simulink model "chris_4R_all_primitives"  (R2024b)
settings: Solver=FixedStepDiscrete  StartTime=0.0  StopTime=60  FixedStep=0.1  MaxStep=0.1  RelTol=1e-3
libraries: neural x220, simulink x1, realtime_pacer_lib x1
(part 1 of 9)
settings Model: Creator=RSL  LastModifiedBy=cwaight
settings SolverCC: AlgebraicLoopSolver=TrustRegion
settings DataIOCC: ReturnWorkspaceOutputs=off
settings DebuggingCC: UnconnectedInputMsg=warning  UnconnectedOutputMsg=warning  UnconnectedLineMsg=warning  ArithmeticOperatorsInVariantConditions=warning
settings ModelReferenceCC: EnableRefExpFcnMdlSchedulingChecks=on
settings SFSimCC: SimUseLocalCustomCode=off  CustomCodeUndefinedFunction=UseInterfaceOnly
settings RTWCC: RTWUseLocalCustomCode=off  GPUComputeCapability=3.5
settings CodeAppCC: StateflowObjectComments=on

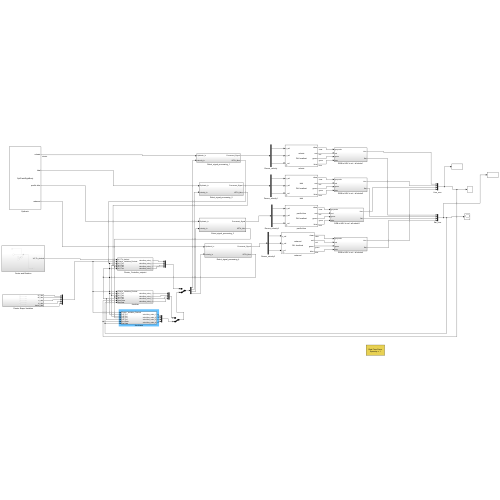
[thumbnail: Simulink's stored preview of the top-level diagram]
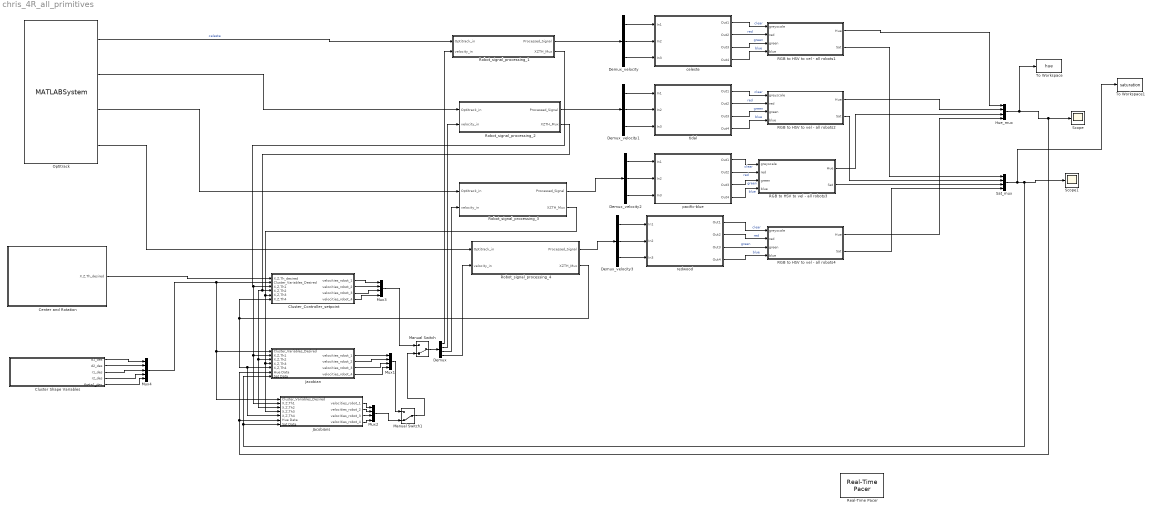
== system chris_4R_all_primitives ==
  Center and Rotation : Subsystem
  Cluster Shape Variables : Subsystem
  Cluster_Controller_setpoint : Subsystem
  Demux : Demux
  Demux_velocity{,1..3} (4 alike) : Demux  Outputs=3
  Hue_mux : Mux
  Jacobian : Subsystem
  Jacobians : Subsystem
  Manual Switch : ManualSwitch  CurrentSetting=0
  Manual Switch1 : ManualSwitch  CurrentSetting=0
  Mux1 : Mux
  Mux2 : Mux
  Mux3 : Mux
  Mux4 : Mux  Inputs=5
  Optitrack : MATLABSystem  System=OptiTrackRigidBody  coordinateTransformationMatrix=[ 1, 0, 0; 0, 0, 1; 0, -1, 0 ]  rigidBodyNames={ 'celeste','tidal','pacific-blue','redwood'}  orientationFormat=Euler angles  debug=on  natNetHostAddress=127.0.0.1  natNetClientAddress=127.0.0.1  dllPath=C:\DecaMATLAB\NatNetSDK\lib\x64\NatNetML.dll  unicast=off
      mask Type: OptiTrackRigidBody
      mask Display:
      | disp('OptiTrackRigidBody');
      | port_label('output',1,'celeste');
      | port_label('output',2,'tidal');
      | port_label('output',3,'pacific-blue');
      | port_label('output',4,'redwood');
  RGB to HSV to vel - all robots1 : Subsystem
  RGB to HSV to vel - all robots2 : Subsystem
  RGB to HSV to vel - all robots3 : Subsystem
  RGB to HSV to vel - all robots4 : Subsystem
  Real-Time Pacer : realtime_pacer_lib/Real-Time Pacer  simTimePerRealTime=1
  Robot_signal_processing_1 : Subsystem
  Robot_signal_processing_2 : Subsystem
  Robot_signal_processing_3 : Subsystem
  Robot_signal_processing_4 : Subsystem
  Sat_mux : Mux
  Scope : Scope
  Scope1 : Scope
  To Workspace : ToWorkspace  VariableName=hue  SaveFormat=Timeseries  SampleTime=-1
  To Workspace1 : ToWorkspace  VariableName=saturation  SaveFormat=Timeseries  SampleTime=-1
  celeste : Subsystem  mask(DecabotMask){robotName=celeste, decabotHelper=localhost, robotAddress=, useDataTurbine=off, useDirectSocket=on, debug=off}
      mask prompts: robotName "Robot name:"; decabotHelper "DecabotHelper/DataTurbine server:"; robotAddress "Robot network address (optional):"; useDataTurbine "Use DataTurbine"; useDirectSocket "Use direct robot TCP connection"; debug "Log debug messages"
      mask help: This is a masked subsystem that contains a Decabot block for bidirectional communication with a decabot over a direct TCP socket connection.
      mask init:
      | robotName = 'Nobody';
      | decabotHelper = 'localhost';
      | robotAddress = '';
      | useDataTurbine = true;
      | debug = true;
      mask TypeOptions robotName: decabot/robotName
      mask Callback robotName:
      | try
      |     set_param( gcb( ), 'Name', get_param( gcb( ), 'robotName' ) );
      | end
      mask TypeOptions decabotHelper: decabot/decabotHelper
      mask TypeOptions robotAddress: decabot/robotAddress
      mask TypeOptions useDataTurbine: decabot/useDataTurbine
      mask TypeOptions useDirectSocket: decabot/useDirectSocket
      mask TypeOptions debug: decabot/debug
      mask Display:
      | disp( [get_param( gcb( ), 'robotName' ) '\n\nDH: ' get_param( gcb( ), 'decabotHelper' ) ] );
      | 
      | port_label('input',1,'x_vel');
      | port_label('input',2,'y_vel');
      | port_label('input',3,'t_vel');
      | 
      | port_label('output',1,'clear');
      | port_label('output',2,'red');
      | port_label('output',3,'green');
      | port_label('output',4,'blue');
  pacific-blue : Subsystem  mask(DecabotMask){robotName=pacific-blue, decabotHelper=localhost, robotAddress=, useDataTurbine=off, useDirectSocket=on, debug=off}
      mask prompts: robotName "Robot name:"; decabotHelper "DecabotHelper/DataTurbine server:"; robotAddress "Robot network address (optional):"; useDataTurbine "Use DataTurbine"; useDirectSocket "Use direct robot TCP connection"; debug "Log debug messages"
      mask help: This is a masked subsystem that contains a Decabot block for bidirectional communication with a decabot over a direct TCP socket connection.
      mask init:
      | robotName = 'Nobody';
      | decabotHelper = 'localhost';
      | robotAddress = '';
      | useDataTurbine = true;
      | debug = true;
      mask TypeOptions robotName: decabot/robotName
      mask Callback robotName:
      | try
      |     set_param( gcb( ), 'Name', get_param( gcb( ), 'robotName' ) );
      | end
      mask TypeOptions decabotHelper: decabot/decabotHelper
      mask TypeOptions robotAddress: decabot/robotAddress
      mask TypeOptions useDataTurbine: decabot/useDataTurbine
      mask TypeOptions useDirectSocket: decabot/useDirectSocket
      mask TypeOptions debug: decabot/debug
      mask Display:
      | disp( [get_param( gcb( ), 'robotName' ) '\n\nDH: ' get_param( gcb( ), 'decabotHelper' ) ] );
      | 
      | port_label('input',1,'x_vel');
      | port_label('input',2,'y_vel');
      | port_label('input',3,'t_vel');
      | 
      | port_label('output',1,'clear');
      | port_label('output',2,'red');
      | port_label('output',3,'green');
      | port_label('output',4,'blue');
  redwood : Subsystem  mask(DecabotMask){robotName=redwood, decabotHelper=localhost, robotAddress=, useDataTurbine=off, useDirectSocket=on, debug=off}
      mask prompts: robotName "Robot name:"; decabotHelper "DecabotHelper/DataTurbine server:"; robotAddress "Robot network address (optional):"; useDataTurbine "Use DataTurbine"; useDirectSocket "Use direct robot TCP connection"; debug "Log debug messages"
      mask help: This is a masked subsystem that contains a Decabot block for bidirectional communication with a decabot over a direct TCP socket connection.
      mask init:
      | robotName = 'Nobody';
      | decabotHelper = 'localhost';
      | robotAddress = '';
      | useDataTurbine = true;
      | debug = true;
      mask TypeOptions robotName: decabot/robotName
      mask Callback robotName:
      | try
      |     set_param( gcb( ), 'Name', get_param( gcb( ), 'robotName' ) );
      | end
      mask TypeOptions decabotHelper: decabot/decabotHelper
      mask TypeOptions robotAddress: decabot/robotAddress
      mask TypeOptions useDataTurbine: decabot/useDataTurbine
      mask TypeOptions useDirectSocket: decabot/useDirectSocket
      mask TypeOptions debug: decabot/debug
      mask Display:
      | disp( [get_param( gcb( ), 'robotName' ) '\n\nDH: ' get_param( gcb( ), 'decabotHelper' ) ] );
      | 
      | port_label('input',1,'x_vel');
      | port_label('input',2,'y_vel');
      | port_label('input',3,'t_vel');
      | 
      | port_label('output',1,'clear');
      | port_label('output',2,'red');
      | port_label('output',3,'green');
      | port_label('output',4,'blue');
  tidal : Subsystem  mask(DecabotMask){robotName=tidal, decabotHelper=localhost, robotAddress=, useDataTurbine=off, useDirectSocket=on, debug=off}
      mask prompts: robotName "Robot name:"; decabotHelper "DecabotHelper/DataTurbine server:"; robotAddress "Robot network address (optional):"; useDataTurbine "Use DataTurbine"; useDirectSocket "Use direct robot TCP connection"; debug "Log debug messages"
      mask help: This is a masked subsystem that contains a Decabot block for bidirectional communication with a decabot over a direct TCP socket connection.
      mask init:
      | robotName = 'Nobody';
      | decabotHelper = 'localhost';
      | robotAddress = '';
      | useDataTurbine = true;
      | debug = true;
      mask TypeOptions robotName: decabot/robotName
      mask Callback robotName:
      | try
      |     set_param( gcb( ), 'Name', get_param( gcb( ), 'robotName' ) );
      | end
      mask TypeOptions decabotHelper: decabot/decabotHelper
      mask TypeOptions robotAddress: decabot/robotAddress
      mask TypeOptions useDataTurbine: decabot/useDataTurbine
      mask TypeOptions useDirectSocket: decabot/useDirectSocket
      mask TypeOptions debug: decabot/debug
      mask Display:
      | disp( [get_param( gcb( ), 'robotName' ) '\n\nDH: ' get_param( gcb( ), 'decabotHelper' ) ] );
      | 
      | port_label('input',1,'x_vel');
      | port_label('input',2,'y_vel');
      | port_label('input',3,'t_vel');
      | 
      | port_label('output',1,'clear');
      | port_label('output',2,'red');
      | port_label('output',3,'green');
      | port_label('output',4,'blue');
  wires:
  Demux_velocity/3 -> celeste/3(In3)
  Demux_velocity/1 -> celeste/1(In1)
  Demux_velocity/2 -> celeste/2(In2)
  Optitrack/1 -> Robot_signal_processing_1/1(Optitrack_in)  "celeste"
  Robot_signal_processing_1/1(Processed_Signal) -> Demux_velocity/1
  Robot_signal_processing_1/2(XZTH_Mux) -> Jacobians/2(X,Z,Th1), Jacobian/2(X,Z,Th1), Cluster_Controller_setpoint/3(X,Z,Th1)
  Demux_velocity1/3 -> tidal/3(In3)
  Demux_velocity1/1 -> tidal/1(In1)
  Demux_velocity1/2 -> tidal/2(In2)
  Robot_signal_processing_2/1(Processed_Signal) -> Demux_velocity1/1
  Demux_velocity2/3 -> pacific-blue/3(In3)
  Demux_velocity2/1 -> pacific-blue/1(In1)
  Demux_velocity2/2 -> pacific-blue/2(In2)
  Robot_signal_processing_3/1(Processed_Signal) -> Demux_velocity2/1
  Robot_signal_processing_3/2(XZTH_Mux) -> Jacobians/4(X,Z,Th3), Jacobian/4(X,Z,Th3), Cluster_Controller_setpoint/5(X,Z,Th3)
  Optitrack/2 -> Robot_signal_processing_2/1(Optitrack_in)
  Cluster_Controller_setpoint/1(velocities_robot_1) -> Mux3/1
  Cluster_Controller_setpoint/3(velocities_robot_3) -> Mux3/3
  Cluster_Controller_setpoint/2(velocities_robot_2) -> Mux3/2
  Mux4/1 -> Jacobian/1(Cluster_Variables_Desired), Jacobians/1(Cluster_Variables_Desired), Cluster_Controller_setpoint/2(Cluster_Variables_Desired)
  Cluster Shape Variables/1(d1_des) -> Mux4/1
  Center and Rotation/1(X,Z,Th_desired) -> Cluster_Controller_setpoint/1(X,Z,Th_desired)
  Demux/1 -> Robot_signal_processing_1/2(velocity_in)
  Demux/2 -> Robot_signal_processing_2/2(velocity_in)
  Demux/3 -> Robot_signal_processing_3/2(velocity_in)
  RGB to HSV to vel - all robots2/1(Hue) -> Hue_mux/2
  RGB to HSV to vel - all robots1/2(Sat) -> Sat_mux/1
  RGB to HSV to vel - all robots1/1(Hue) -> Hue_mux/1
  Cluster Shape Variables/2(d2_des) -> Mux4/2
  Hue_mux/1 -> To Workspace/1, Jacobians/6(Hue Data), Jacobian/6(Hue Data), Scope/1
  Sat_mux/1 -> To Workspace1/1, Jacobians/7(Sat Data), Jacobian/7(Sat Data), Scope1/1
  Demux/4 -> Robot_signal_processing_4/2(velocity_in)
  Robot_signal_processing_4/2(XZTH_Mux) -> Jacobians/5(X,Z,Th4), Jacobian/5(X,Z,Th4), Cluster_Controller_setpoint/6(X,Z,Th4)
  Demux_velocity3/2 -> redwood/2(In2)
  Demux_velocity3/3 -> redwood/3(In3)
  Demux_velocity3/1 -> redwood/1(In1)
  Robot_signal_processing_4/1(Processed_Signal) -> Demux_velocity3/1
  RGB to HSV to vel - all robots4/1(Hue) -> Hue_mux/4
  RGB to HSV to vel - all robots4/2(Sat) -> Sat_mux/4
  Cluster Shape Variables/3(r1_des) -> Mux4/3
  Cluster Shape Variables/4(r2_des) -> Mux4/4
  Cluster Shape Variables/5(theta1_des) -> Mux4/5
  Cluster_Controller_setpoint/4(velocities_robot_4) -> Mux3/4
  celeste/1(Out1) -> RGB to HSV to vel - all robots1/1(greyscale)  "clear"
  celeste/2(Out2) -> RGB to HSV to vel - all robots1/2(red)  "red"
  celeste/3(Out3) -> RGB to HSV to vel - all robots1/3(green)  "green"
  celeste/4(Out4) -> RGB to HSV to vel - all robots1/4(blue)  "blue"
  tidal/1(Out1) -> RGB to HSV to vel - all robots2/1(greyscale)  "clear"
  tidal/2(Out2) -> RGB to HSV to vel - all robots2/2(red)  "red"
  tidal/3(Out3) -> RGB to HSV to vel - all robots2/3(green)  "green"
  tidal/4(Out4) -> RGB to HSV to vel - all robots2/4(blue)  "blue"
  pacific-blue/1(Out1) -> RGB to HSV to vel - all robots3/1(greyscale)  "clear"
  pacific-blue/2(Out2) -> RGB to HSV to vel - all robots3/2(red)  "red"
  pacific-blue/3(Out3) -> RGB to HSV to vel - all robots3/3(green)  "green"
  pacific-blue/4(Out4) -> RGB to HSV to vel - all robots3/4(blue)  "blue"
  redwood/1(Out1) -> RGB to HSV to vel - all robots4/1(greyscale)  "clear"
  redwood/2(Out2) -> RGB to HSV to vel - all robots4/2(red)  "red"
  redwood/3(Out3) -> RGB to HSV to vel - all robots4/3(green)  "green"
  redwood/4(Out4) -> RGB to HSV to vel - all robots4/4(blue)  "blue"
  Jacobian/1(velocities_robot_1) -> Mux1/1
  Jacobian/2(velocities_robot_2) -> Mux1/2
  Jacobian/3(velocities_robot_3) -> Mux1/3
  Jacobian/4(velocities_robot_4) -> Mux1/4
  Mux3/1 -> Manual Switch/1
  Manual Switch/1 -> Demux/1
  Optitrack/3 -> Robot_signal_processing_3/1(Optitrack_in)
  Optitrack/4 -> Robot_signal_processing_4/1(Optitrack_in)
  Manual Switch1/1 -> Manual Switch/2
  Mux1/1 -> Manual Switch1/1
  Mux2/1 -> Manual Switch1/2
  Jacobians/1(velocities_robot_1) -> Mux2/1
  Jacobians/2(velocities_robot_2) -> Mux2/2
  Jacobians/3(velocities_robot_3) -> Mux2/3
  Jacobians/4(velocities_robot_4) -> Mux2/4
  Robot_signal_processing_2/2(XZTH_Mux) -> Jacobians/3(X,Z,Th2), Jacobian/3(X,Z,Th2), Cluster_Controller_setpoint/4(X,Z,Th2)
  RGB to HSV to vel - all robots3/1(Hue) -> Hue_mux/3
  RGB to HSV to vel - all robots3/2(Sat) -> Sat_mux/3
  RGB to HSV to vel - all robots2/2(Sat) -> Sat_mux/2

== system chris_4R_all_primitives/Center and Rotation ==
  Manual Switch : ManualSwitch
  Mux3 : Mux  Inputs=3
  Ramp : simulink/Sources/Ramp  slope=0.1  start=0  InitialOutput=0
  "Theta_Set Point1 " : Constant  Value=-pi/2
  xc : Constant  Value=0
  yc : Constant  Value=0
  X,Z,Th_desired : Outport
  wires:
  Mux3/1 -> X,Z,Th_desired/1
  Manual Switch/1 -> Mux3/3
  Ramp/1 -> Manual Switch/2
  xc/1 -> Mux3/1
  yc/1 -> Mux3/2
  "Theta_Set Point1 "/1 -> Manual Switch/1

== system chris_4R_all_primitives/Cluster Shape Variables ==
  Theta1 : Constant  Value=pi/2
  d1 : Constant  Value=0.25
  d2 : Constant  Value=0.433
  r1 : Constant  Value=.5
  r2 : Constant  Value=.5
  d1_des : Outport
  d2_des : Outport  Port=2
  r1_des : Outport  Port=3
  r2_des : Outport  Port=4
  theta1_des : Outport  Port=5
  wires:
  d1/1 -> d1_des/1
  Theta1/1 -> theta1_des/1
  d2/1 -> d2_des/1
  r1/1 -> r1_des/1
  r2/1 -> r2_des/1

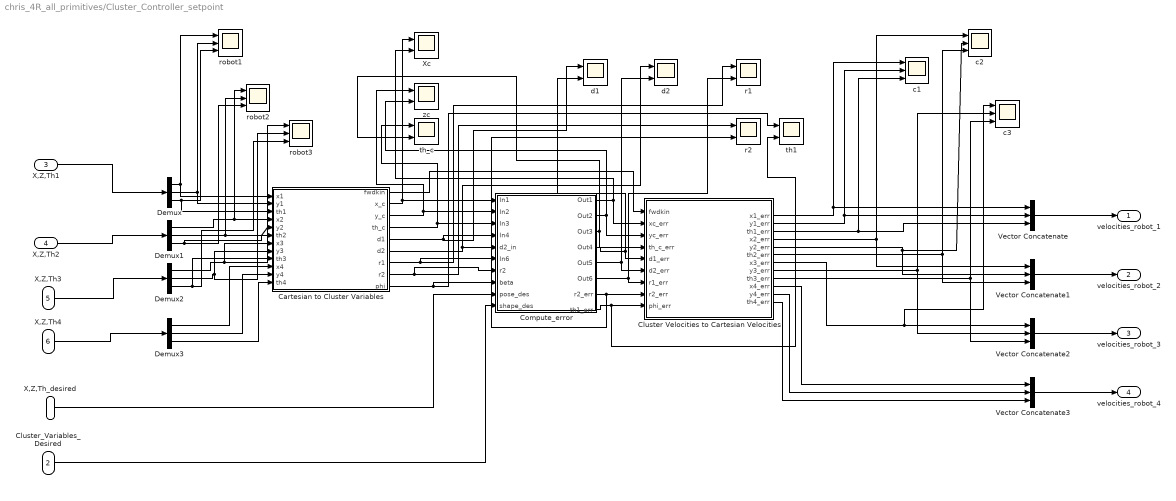
== system chris_4R_all_primitives/Cluster_Controller_setpoint ==
  X,Z,Th_desired : Inport
  Cluster_Variables_Desired : Inport  Port=2
  X,Z,Th1 : Inport  Port=3
  X,Z,Th2 : Inport  Port=4
  X,Z,Th3 : Inport  Port=5
  X,Z,Th4 : Inport  Port=6
  Cartesian to Cluster Variables : MATLAB Function  TreatAsAtomicUnit=on
  Cluster Velocities to Cartesian Velocities : MATLAB Function  TreatAsAtomicUnit=on
  Compute_error : Subsystem
  Demux{,1..3} (4 alike) : Demux  Outputs=3
  Vector Concatenate{,1..3} (4 alike) : Concatenate  NumInputs=3
  Xc : Scope  NumInputPorts=2
  c1 : Scope  NumInputPorts=3
  c2 : Scope  NumInputPorts=3
  c3 : Scope  NumInputPorts=3
  d1 : Scope  NumInputPorts=2
  d2 : Scope  NumInputPorts=2
  r1 : Scope  NumInputPorts=2
  r2 : Scope  NumInputPorts=2
  robot1 : Scope  NumInputPorts=3
  robot2 : Scope  NumInputPorts=3
  robot3 : Scope  NumInputPorts=3
  th1 : Scope  NumInputPorts=2
  th_c : Scope  NumInputPorts=2
  zc : Scope  NumInputPorts=2
  velocities_robot_1 : Outport
  velocities_robot_2 : Outport  Port=2
  velocities_robot_3 : Outport  Port=3
  velocities_robot_4 : Outport  Port=4
  wires:
  X,Z,Th1/1 -> Demux/1
  X,Z,Th2/1 -> Demux1/1
  X,Z,Th3/1 -> Demux2/1
  Vector Concatenate/1 -> velocities_robot_1/1
  Cluster Velocities to Cartesian Velocities/2(y1_err) -> c1/2, Vector Concatenate/2
  Cluster Velocities to Cartesian Velocities/1(x1_err) -> c1/1, Vector Concatenate/1
  Vector Concatenate1/1 -> velocities_robot_2/1
  Cluster Velocities to Cartesian Velocities/5(y2_err) -> Vector Concatenate1/2, c2/2
  Cluster Velocities to Cartesian Velocities/4(x2_err) -> Vector Concatenate1/1, c2/1
  Vector Concatenate2/1 -> velocities_robot_3/1
  Cluster Velocities to Cartesian Velocities/8(y3_err) -> Vector Concatenate2/2, c3/2
  Cluster Velocities to Cartesian Velocities/7(x3_err) -> c3/1, Vector Concatenate2/1
  Demux/1 -> robot1/1, Cartesian to Cluster Variables/1(x1)
  Demux/2 -> robot1/2, Cartesian to Cluster Variables/2(y1)
  Demux/3 -> Cartesian to Cluster Variables/3(th1), robot1/3
  Demux1/1 -> robot2/1, Cartesian to Cluster Variables/4(x2)
  Demux1/2 -> robot2/2, Cartesian to Cluster Variables/5(y2)
  Demux1/3 -> Cartesian to Cluster Variables/6(th2), robot2/3
  Demux2/1 -> robot3/1, Cartesian to Cluster Variables/7(x3)
  Demux2/2 -> robot3/2, Cartesian to Cluster Variables/8(y3)
  Demux2/3 -> Cartesian to Cluster Variables/9(th3), robot3/3
  Cartesian to Cluster Variables/2(x_c) -> Xc/1, Compute_error/1(In1)
  Cartesian to Cluster Variables/3(y_c) -> zc/1, Compute_error/2(In2)
  Cartesian to Cluster Variables/4(th_c) -> Compute_error/3(In3), th_c/1
  Cartesian to Cluster Variables/5(d1) -> d1/1, Compute_error/4(In4)
  Cartesian to Cluster Variables/6(d2) -> Compute_error/5(d2_in), d2/1
  Cartesian to Cluster Variables/7(r1) -> r1/1, Compute_error/6(In6)
  X,Z,Th_desired/1 -> Compute_error/9(pose_des)
  Cluster_Variables_Desired/1 -> Compute_error/10(shape_des)
  Compute_error/1(Out1) -> Cluster Velocities to Cartesian Velocities/2(xc_err), Xc/2
  Compute_error/2(Out2) -> Cluster Velocities to Cartesian Velocities/3(yc_err), zc/2
  Compute_error/3(Out3) -> Cluster Velocities to Cartesian Velocities/4(th_c_err), th_c/2
  Compute_error/4(Out4) -> Cluster Velocities to Cartesian Velocities/5(d1_err), d1/2
  Compute_error/5(Out5) -> Cluster Velocities to Cartesian Velocities/6(d2_err), d2/2
  Compute_error/6(Out6) -> Cluster Velocities to Cartesian Velocities/7(r1_err), r1/2
  Cartesian to Cluster Variables/1(fwdkin) -> Cluster Velocities to Cartesian Velocities/1(fwdkin)
  Cluster Velocities to Cartesian Velocities/3(th1_err) -> c1/3, Vector Concatenate/3
  Cluster Velocities to Cartesian Velocities/6(th2_err) -> Vector Concatenate1/3, c2/3
  Cluster Velocities to Cartesian Velocities/9(th3_err) -> Vector Concatenate2/3, c3/3
  Vector Concatenate3/1 -> velocities_robot_4/1
  X,Z,Th4/1 -> Demux3/1
  Demux3/1 -> Cartesian to Cluster Variables/10(x4)
  Demux3/2 -> Cartesian to Cluster Variables/11(y4)
  Cartesian to Cluster Variables/8(r2) -> r2/1, Compute_error/7(r2)
  Cartesian to Cluster Variables/9(phi) -> th1/1, Compute_error/8(beta)
  Compute_error/7(r2_err) -> Cluster Velocities to Cartesian Velocities/8(r2_err), r2/2
  Compute_error/8(th1_err) -> th1/2, Cluster Velocities to Cartesian Velocities/9(phi_err)
  Cluster Velocities to Cartesian Velocities/10(x4_err) -> Vector Concatenate3/1
  Cluster Velocities to Cartesian Velocities/11(y4_err) -> Vector Concatenate3/2
  Cluster Velocities to Cartesian Velocities/12(th4_err) -> Vector Concatenate3/3
  Demux3/3 -> Cartesian to Cluster Variables/12(th4)

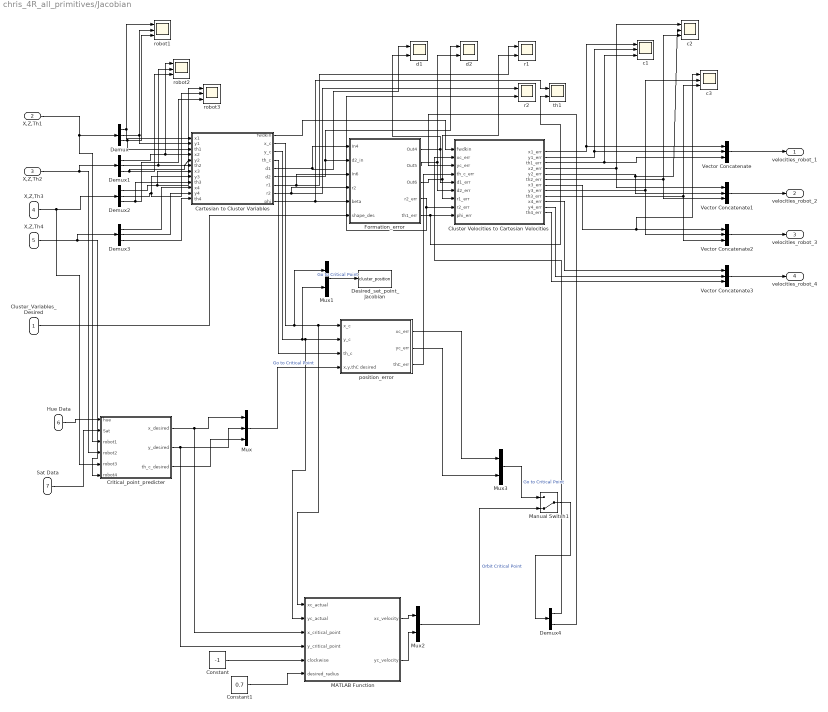
== system chris_4R_all_primitives/Jacobian ==
  Cluster_Variables_Desired : Inport
  X,Z,Th1 : Inport  Port=2
  X,Z,Th2 : Inport  Port=3
  X,Z,Th3 : Inport  Port=4
  X,Z,Th4 : Inport  Port=5
  Hue Data : Inport  Port=6
  Sat Data : Inport  Port=7
  Cartesian to Cluster Variables : MATLAB Function  TreatAsAtomicUnit=on
  Cluster Velocities to Cartesian Velocities : MATLAB Function  TreatAsAtomicUnit=on
  Constant : Constant  Value=-1
  Constant1 : Constant  Value=0.7
  Critical_point_predicter : Subsystem
  Demux{,1..3} (4 alike) : Demux  Outputs=3
  Demux4 : Demux  Outputs=2
  Desired_set_point_Jacobian : ToWorkspace  VariableName=cluster_position  SampleTime=-1
  Formation_error : Subsystem
  MATLAB Function : MATLAB Function  TreatAsAtomicUnit=on
  Manual Switch1 : ManualSwitch  CurrentSetting=0
  Mux : Mux  Inputs=3
  Mux1 : Mux  Inputs=2
  Mux2 : Mux  Inputs=2
  Mux3 : Mux  Inputs=2
  Vector Concatenate{,1..3} (4 alike) : Concatenate  NumInputs=3
  c1 : Scope  NumInputPorts=3
  c2 : Scope  NumInputPorts=3
  c3 : Scope  NumInputPorts=3
  d1 : Scope  NumInputPorts=2
  d2 : Scope  NumInputPorts=2
  position_error : Subsystem
  r1 : Scope  NumInputPorts=2
  r2 : Scope  NumInputPorts=2
  robot1 : Scope  NumInputPorts=3
  robot2 : Scope  NumInputPorts=3
  robot3 : Scope  NumInputPorts=3
  th1 : Scope  NumInputPorts=2
  velocities_robot_1 : Outport
  velocities_robot_2 : Outport  Port=2
  velocities_robot_3 : Outport  Port=3
  velocities_robot_4 : Outport  Port=4
  wires:
  X,Z,Th1/1 -> Critical_point_predicter/3(robot1), Demux/1
  X,Z,Th2/1 -> Critical_point_predicter/4(robot2), Demux1/1
  X,Z,Th3/1 -> Critical_point_predicter/5(robot3), Demux2/1
  Vector Concatenate/1 -> velocities_robot_1/1
  Cluster Velocities to Cartesian Velocities/2(y1_err) -> c1/2, Vector Concatenate/2
  Cluster Velocities to Cartesian Velocities/1(x1_err) -> c1/1, Vector Concatenate/1
  Vector Concatenate1/1 -> velocities_robot_2/1
  Cluster Velocities to Cartesian Velocities/5(y2_err) -> Vector Concatenate1/2, c2/2
  Cluster Velocities to Cartesian Velocities/4(x2_err) -> Vector Concatenate1/1, c2/1
  Vector Concatenate2/1 -> velocities_robot_3/1
  Cluster Velocities to Cartesian Velocities/8(y3_err) -> Vector Concatenate2/2, c3/2
  Cluster Velocities to Cartesian Velocities/7(x3_err) -> c3/1, Vector Concatenate2/1
  Demux/1 -> robot1/1, Cartesian to Cluster Variables/1(x1)
  Demux/2 -> robot1/2, Cartesian to Cluster Variables/2(y1)
  Demux/3 -> Cartesian to Cluster Variables/3(th1), robot1/3
  Demux1/1 -> robot2/1, Cartesian to Cluster Variables/4(x2)
  Demux1/2 -> robot2/2, Cartesian to Cluster Variables/5(y2)
  Demux1/3 -> Cartesian to Cluster Variables/6(th2), robot2/3
  Demux2/1 -> robot3/1, Cartesian to Cluster Variables/7(x3)
  Demux2/2 -> robot3/2, Cartesian to Cluster Variables/8(y3)
  Demux2/3 -> Cartesian to Cluster Variables/9(th3), robot3/3
  Cartesian to Cluster Variables/5(d1) -> d1/1, Formation_error/1(In4)
  Cartesian to Cluster Variables/6(d2) -> d2/1, Formation_error/2(d2_in)
  Cartesian to Cluster Variables/7(r1) -> r1/1, Formation_error/3(In6)
  Cluster_Variables_Desired/1 -> Formation_error/6(shape_des)
  Formation_error/1(Out4) -> d1/2, Cluster Velocities to Cartesian Velocities/5(d1_err)
  Formation_error/2(Out5) -> Cluster Velocities to Cartesian Velocities/6(d2_err), d2/2
  Formation_error/3(Out6) -> Cluster Velocities to Cartesian Velocities/7(r1_err), r1/2
  Cartesian to Cluster Variables/1(fwdkin) -> Cluster Velocities to Cartesian Velocities/1(fwdkin)
  Cluster Velocities to Cartesian Velocities/3(th1_err) -> c1/3, Vector Concatenate/3
  Cluster Velocities to Cartesian Velocities/6(th2_err) -> Vector Concatenate1/3, c2/3
  Cluster Velocities to Cartesian Velocities/9(th3_err) -> Vector Concatenate2/3, c3/3
  Vector Concatenate3/1 -> velocities_robot_4/1
  X,Z,Th4/1 -> Critical_point_predicter/6(robot4), Demux3/1
  Demux3/1 -> Cartesian to Cluster Variables/10(x4)
  Demux3/2 -> Cartesian to Cluster Variables/11(y4)
  Cartesian to Cluster Variables/8(r2) -> r2/1, Formation_error/4(r2)
  Cartesian to Cluster Variables/9(phi) -> th1/1, Formation_error/5(beta)
  Formation_error/4(r2_err) -> Cluster Velocities to Cartesian Velocities/8(r2_err), r2/2
  Formation_error/5(th1_err) -> th1/2, Cluster Velocities to Cartesian Velocities/9(phi_err)
  Cluster Velocities to Cartesian Velocities/10(x4_err) -> Vector Concatenate3/1
  Cluster Velocities to Cartesian Velocities/11(y4_err) -> Vector Concatenate3/2
  Cluster Velocities to Cartesian Velocities/12(th4_err) -> Vector Concatenate3/3
  Demux3/3 -> Cartesian to Cluster Variables/12(th4)
  Cartesian to Cluster Variables/4(th_c) -> position_error/3(th_c)
  position_error/3(thC_err) -> Cluster Velocities to Cartesian Velocities/4(th_c_err)
  Cartesian to Cluster Variables/2(x_c) -> Mux1/1, MATLAB Function/1(xc_actual), position_error/1(x_c)
  Constant1/1 -> MATLAB Function/6(desired_radius)
  Cartesian to Cluster Variables/3(y_c) -> Mux1/2, MATLAB Function/2(yc_actual), position_error/2(y_c)
  Constant/1 -> MATLAB Function/5(clockwise)
  MATLAB Function/1(xc_velocity) -> Mux2/1
  MATLAB Function/2(yc_velocity) -> Mux2/2
  Hue Data/1 -> Critical_point_predicter/1(hue)
  Sat Data/1 -> Critical_point_predicter/2(Sat)
  Critical_point_predicter/3(th_c_desired) -> Mux/3
  Mux/1 -> position_error/4(x,y,thC desired)  "Go to Critical Point"
  Critical_point_predicter/1(x_desired) -> MATLAB Function/3(x_critical_point), Mux/1
  Critical_point_predicter/2(y_desired) -> MATLAB Function/4(y_critical_point), Mux/2
  Mux3/1 -> Manual Switch1/1  "Go to Critical Point"
  Mux2/1 -> Manual Switch1/2  "Orbit Critical Point"
  position_error/1(xc_err) -> Mux3/1
  position_error/2(yc_err) -> Mux3/2
  Manual Switch1/1 -> Demux4/1
  Demux4/1 -> Cluster Velocities to Cartesian Velocities/2(xc_err)
  Demux4/2 -> Cluster Velocities to Cartesian Velocities/3(yc_err)
  Mux1/1 -> Desired_set_point_Jacobian/1  "Go to Critical Point"

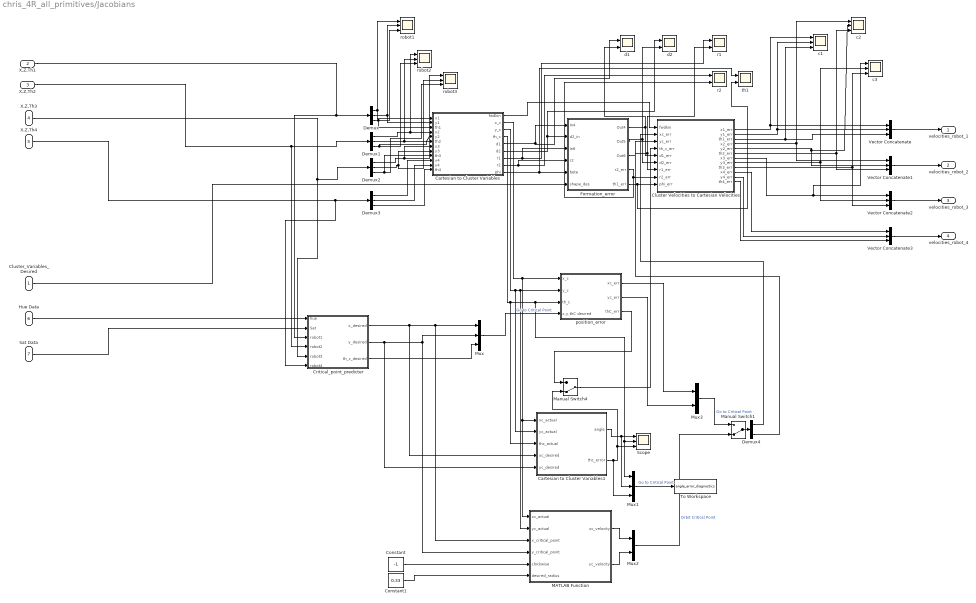
== system chris_4R_all_primitives/Jacobians ==
  Cluster_Variables_Desired : Inport
  X,Z,Th1 : Inport  Port=2
  X,Z,Th2 : Inport  Port=3
  X,Z,Th3 : Inport  Port=4
  X,Z,Th4 : Inport  Port=5
  Hue Data : Inport  Port=6
  Sat Data : Inport  Port=7
  Cartesian to Cluster Variables : MATLAB Function  TreatAsAtomicUnit=on
  Cartesian to Cluster Variables1 : MATLAB Function  TreatAsAtomicUnit=on
  Cluster Velocities to Cartesian Velocities : MATLAB Function  TreatAsAtomicUnit=on
  Constant : Constant  Value=-1
  Constant1 : Constant  Value=0.33
  Critical_point_predicter : Subsystem
  Demux{,1..3} (4 alike) : Demux  Outputs=3
  Demux4 : Demux  Outputs=2
  Formation_error : Subsystem
  MATLAB Function : MATLAB Function  TreatAsAtomicUnit=on
  Manual Switch1 : ManualSwitch  CurrentSetting=0
  Manual Switch4 : ManualSwitch  CurrentSetting=0
  Mux : Mux  Inputs=3
  Mux1 : Mux  Inputs=3
  Mux2 : Mux  Inputs=2
  Mux3 : Mux  Inputs=2
  Scope : Scope  NumInputPorts=3
  To Workspace : ToWorkspace  VariableName=angle_error_diagnostics  SaveFormat=Timeseries  SampleTime=-1
  Vector Concatenate{,1..3} (4 alike) : Concatenate  NumInputs=3
  c1 : Scope  NumInputPorts=3
  c2 : Scope  NumInputPorts=3
  c3 : Scope  NumInputPorts=3
  d1 : Scope  NumInputPorts=2
  d2 : Scope  NumInputPorts=2
  position_error : Subsystem
  r1 : Scope  NumInputPorts=2
  r2 : Scope  NumInputPorts=2
  robot1 : Scope  NumInputPorts=3
  robot2 : Scope  NumInputPorts=3
  robot3 : Scope  NumInputPorts=3
  th1 : Scope  NumInputPorts=2
  velocities_robot_1 : Outport
  velocities_robot_2 : Outport  Port=2
  velocities_robot_3 : Outport  Port=3
  velocities_robot_4 : Outport  Port=4
  wires:
  X,Z,Th1/1 -> Critical_point_predicter/3(robot1), Demux/1
  X,Z,Th2/1 -> Demux1/1, Critical_point_predicter/4(robot2)
  X,Z,Th3/1 -> Critical_point_predicter/5(robot3), Demux2/1
  Vector Concatenate/1 -> velocities_robot_1/1
  Cluster Velocities to Cartesian Velocities/2(y1_err) -> c1/2, Vector Concatenate/2
  Cluster Velocities to Cartesian Velocities/1(x1_err) -> c1/1, Vector Concatenate/1
  Vector Concatenate1/1 -> velocities_robot_2/1
  Cluster Velocities to Cartesian Velocities/5(y2_err) -> Vector Concatenate1/2, c2/2
  Cluster Velocities to Cartesian Velocities/4(x2_err) -> Vector Concatenate1/1, c2/1
  Vector Concatenate2/1 -> velocities_robot_3/1
  Cluster Velocities to Cartesian Velocities/8(y3_err) -> Vector Concatenate2/2, c3/2
  Cluster Velocities to Cartesian Velocities/7(x3_err) -> c3/1, Vector Concatenate2/1
  Demux/1 -> robot1/1, Cartesian to Cluster Variables/1(x1)
  Demux/2 -> robot1/2, Cartesian to Cluster Variables/2(y1)
  Demux/3 -> Cartesian to Cluster Variables/3(th1), robot1/3
  Demux1/1 -> robot2/1, Cartesian to Cluster Variables/4(x2)
  Demux1/2 -> robot2/2, Cartesian to Cluster Variables/5(y2)
  Demux1/3 -> Cartesian to Cluster Variables/6(th2), robot2/3
  Demux2/1 -> robot3/1, Cartesian to Cluster Variables/7(x3)
  Demux2/2 -> robot3/2, Cartesian to Cluster Variables/8(y3)
  Demux2/3 -> Cartesian to Cluster Variables/9(th3), robot3/3
  Cartesian to Cluster Variables/5(d1) -> d1/1, Formation_error/1(In4)
  Cartesian to Cluster Variables/6(d2) -> d2/1, Formation_error/2(d2_in)
  Cartesian to Cluster Variables/7(r1) -> r1/1, Formation_error/3(In6)
  Cluster_Variables_Desired/1 -> Formation_error/6(shape_des)
  Formation_error/1(Out4) -> d1/2, Cluster Velocities to Cartesian Velocities/5(d1_err)
  Formation_error/2(Out5) -> Cluster Velocities to Cartesian Velocities/6(d2_err), d2/2
  Formation_error/3(Out6) -> Cluster Velocities to Cartesian Velocities/7(r1_err), r1/2
  Cartesian to Cluster Variables/1(fwdkin) -> Cluster Velocities to Cartesian Velocities/1(fwdkin)
  Cluster Velocities to Cartesian Velocities/3(th1_err) -> c1/3, Vector Concatenate/3
  Cluster Velocities to Cartesian Velocities/6(th2_err) -> Vector Concatenate1/3, c2/3
  Cluster Velocities to Cartesian Velocities/9(th3_err) -> Vector Concatenate2/3, c3/3
  Vector Concatenate3/1 -> velocities_robot_4/1
  X,Z,Th4/1 -> Critical_point_predicter/6(robot4), Demux3/1
  Demux3/1 -> Cartesian to Cluster Variables/10(x4)
  Demux3/2 -> Cartesian to Cluster Variables/11(y4)
  Cartesian to Cluster Variables/8(r2) -> r2/1, Formation_error/4(r2)
  Cartesian to Cluster Variables/9(phi) -> th1/1, Formation_error/5(beta)
  Formation_error/4(r2_err) -> Cluster Velocities to Cartesian Velocities/8(r2_err), r2/2
  Formation_error/5(th1_err) -> th1/2, Cluster Velocities to Cartesian Velocities/9(phi_err)
  Cluster Velocities to Cartesian Velocities/10(x4_err) -> Vector Concatenate3/1
  Cluster Velocities to Cartesian Velocities/11(y4_err) -> Vector Concatenate3/2
  Cluster Velocities to Cartesian Velocities/12(th4_err) -> Vector Concatenate3/3
  Demux3/3 -> Cartesian to Cluster Variables/12(th4)
  Cartesian to Cluster Variables/4(th_c) -> Cartesian to Cluster Variables1/3(thc_actual), Mux1/1, Scope/2, position_error/3(th_c)
  Cartesian to Cluster Variables/2(x_c) -> position_error/1(x_c), Cartesian to Cluster Variables1/1(xc_actual), MATLAB Function/1(xc_actual)
  Constant1/1 -> MATLAB Function/6(desired_radius)
  Cartesian to Cluster Variables/3(y_c) -> Cartesian to Cluster Variables1/2(yc_actual), MATLAB Function/2(yc_actual), position_error/2(y_c)
  Constant/1 -> MATLAB Function/5(clockwise)
  MATLAB Function/1(xc_velocity) -> Mux2/1
  MATLAB Function/2(yc_velocity) -> Mux2/2
  Hue Data/1 -> Critical_point_predicter/1(hue)
  Sat Data/1 -> Critical_point_predicter/2(Sat)
  Critical_point_predicter/3(th_c_desired) -> Mux/3
  Mux/1 -> position_error/4(x,y,thC desired)  "Go to Critical Point"
  Critical_point_predicter/1(x_desired) -> Cartesian to Cluster Variables1/4(xc_desired), MATLAB Function/3(x_critical_point), Mux/1
  Critical_point_predicter/2(y_desired) -> Cartesian to Cluster Variables1/5(yc_desired), MATLAB Function/4(y_critical_point), Mux/2
  Mux3/1 -> Manual Switch1/1  "Go to Critical Point"
  Mux2/1 -> Manual Switch1/2  "Orbit Critical Point"
  position_error/1(xc_err) -> Mux3/1
  position_error/2(yc_err) -> Mux3/2
  Manual Switch1/1 -> Demux4/1
  Demux4/1 -> Cluster Velocities to Cartesian Velocities/2(xc_err)
  Demux4/2 -> Cluster Velocities to Cartesian Velocities/3(yc_err)
  position_error/3(thC_err) -> Manual Switch4/1
  Manual Switch4/1 -> Cluster Velocities to Cartesian Velocities/4(th_c_err)
  Cartesian to Cluster Variables1/2(thc_error) -> Mux1/3, Scope/3, Manual Switch4/2
  Cartesian to Cluster Variables1/1(angle) -> Mux1/2, Scope/1
  Mux1/1 -> To Workspace/1  "Go to Critical Point"

== system chris_4R_all_primitives/RGB to HSV to vel - all robots1 ==
  greyscale : Inport
  red : Inport  Port=2
  green : Inport  Port=3
  blue : Inport  Port=4
  B : Display
  Demux : Demux  Outputs=2
  G : Display
  Hue Neural Network : Subsystem
      mask help: Feed-Forward Neural Network
      mask Display: e = 0.06;c1 = [120 150 230]/255;c2 = ([120 150 230]+0)/383;c3 = ([120 150 230]+128)/383;patch([0 1 1 0],[0 0 1 1],c1);patch([0 1 1 1-e 1-e 0+e],[0 0 1 1-e 0+e 0+e],c2);patch([0 0 1 1-e 0+e 0+e],[0 1 1 1-e 1-e 0+e],c3);plot([0 1 1 0 0],[0 0 1 1 0]);fprintf('NNET');port_label('input',1,' Input');port_label('output',1,'Output ');
  Hue_adjusted : Display
  K : Display
  Mux : Mux
  R : Display
  RGB to HSV : MATLAB Function  TreatAsAtomicUnit=on
  Sat Neural Network : Subsystem
      mask help: Feed-Forward Neural Network
      mask Display: e = 0.06;c1 = [120 150 230]/255;c2 = ([120 150 230]+0)/383;c3 = ([120 150 230]+128)/383;patch([0 1 1 0],[0 0 1 1],c1);patch([0 1 1 1-e 1-e 0+e],[0 0 1 1-e 0+e 0+e],c2);patch([0 0 1 1-e 0+e 0+e],[0 1 1 1-e 1-e 0+e],c3);plot([0 1 1 0 0],[0 0 1 1 0]);fprintf('NNET');port_label('input',1,' Input');port_label('output',1,'Output ');
  Saturation_adjusted : Display
  hue_post_processor : MATLAB Function  TreatAsAtomicUnit=on
  sat_post_processor : MATLAB Function  TreatAsAtomicUnit=on
  sat_post_processor1 : MATLAB Function  TreatAsAtomicUnit=on
  Hue : Outport
  Sat : Outport  Port=2
  wires:
  red/1 -> R/1, RGB to HSV/1("R ")  "red"
  green/1 -> G/1, RGB to HSV/2("G ")  "green"
  blue/1 -> B/1, RGB to HSV/3("B ")  "blue"
  greyscale/1 -> K/1, RGB to HSV/4("K ")
  RGB to HSV/4(K) -> Mux/4
  RGB to HSV/3(B) -> Mux/3
  RGB to HSV/2(G) -> Mux/2
  RGB to HSV/1(R) -> Mux/1
  hue_post_processor/1(hue) -> Hue_adjusted/1, Hue/1
  sat_post_processor/1(sat) -> Sat/1, Saturation_adjusted/1
  Hue Neural Network/1(Output) -> Demux/1
  Demux/1 -> hue_post_processor/1(hue_nn_sin)
  Demux/2 -> hue_post_processor/2(hue_nn_cos)
  sat_post_processor1/1(data) -> Hue Neural Network/1(Input), Sat Neural Network/1(Input)
  Mux/1 -> sat_post_processor1/1(data_raw)
  Sat Neural Network/1(Output) -> sat_post_processor/1(sat_nn_output)

== system chris_4R_all_primitives/RGB to HSV to vel - all robots2 ==
  greyscale : Inport
  red : Inport  Port=2
  green : Inport  Port=3
  blue : Inport  Port=4
  B : Display
  Demux : Demux  Outputs=2
  G : Display
  Hue Neural Network : Subsystem
      mask help: Feed-Forward Neural Network
      mask Display: e = 0.06;c1 = [120 150 230]/255;c2 = ([120 150 230]+0)/383;c3 = ([120 150 230]+128)/383;patch([0 1 1 0],[0 0 1 1],c1);patch([0 1 1 1-e 1-e 0+e],[0 0 1 1-e 0+e 0+e],c2);patch([0 0 1 1-e 0+e 0+e],[0 1 1 1-e 1-e 0+e],c3);plot([0 1 1 0 0],[0 0 1 1 0]);fprintf('NNET');port_label('input',1,' Input');port_label('output',1,'Output ');
  Hue_adjusted : Display
  K : Display
  Mux : Mux
  R : Display
  RGB to HSV : MATLAB Function  TreatAsAtomicUnit=on
  Sat Neural Network : Subsystem
      mask help: Feed-Forward Neural Network
      mask Display: e = 0.06;c1 = [120 150 230]/255;c2 = ([120 150 230]+0)/383;c3 = ([120 150 230]+128)/383;patch([0 1 1 0],[0 0 1 1],c1);patch([0 1 1 1-e 1-e 0+e],[0 0 1 1-e 0+e 0+e],c2);patch([0 0 1 1-e 0+e 0+e],[0 1 1 1-e 1-e 0+e],c3);plot([0 1 1 0 0],[0 0 1 1 0]);fprintf('NNET');port_label('input',1,' Input');port_label('output',1,'Output ');
  Saturation_adjusted : Display
  hue_post_processor : MATLAB Function  TreatAsAtomicUnit=on
  sat_post_processor : MATLAB Function  TreatAsAtomicUnit=on
  sat_post_processor1 : MATLAB Function  TreatAsAtomicUnit=on
  Hue : Outport
  Sat : Outport  Port=2
  wires:
  red/1 -> R/1, RGB to HSV/1("R ")  "red"
  green/1 -> G/1, RGB to HSV/2("G ")  "green"
  blue/1 -> B/1, RGB to HSV/3("B ")  "blue"
  greyscale/1 -> K/1, RGB to HSV/4("K ")
  RGB to HSV/4(K) -> Mux/4
  RGB to HSV/3(B) -> Mux/3
  RGB to HSV/2(G) -> Mux/2
  RGB to HSV/1(R) -> Mux/1
  hue_post_processor/1(hue) -> Hue_adjusted/1, Hue/1
  sat_post_processor/1(sat) -> Sat/1, Saturation_adjusted/1
  Hue Neural Network/1(Output) -> Demux/1
  Demux/1 -> hue_post_processor/1(hue_nn_sin)
  Demux/2 -> hue_post_processor/2(hue_nn_cos)
  sat_post_processor1/1(data) -> Hue Neural Network/1(Input), Sat Neural Network/1(Input)
  Mux/1 -> sat_post_processor1/1(data_raw)
  Sat Neural Network/1(Output) -> sat_post_processor/1(sat_nn_output)

== system chris_4R_all_primitives/RGB to HSV to vel - all robots3 ==
  greyscale : Inport
  red : Inport  Port=2
  green : Inport  Port=3
  blue : Inport  Port=4
  B : Display
  Demux : Demux  Outputs=2
  G : Display
  Hue Neural Network : Subsystem
      mask help: Feed-Forward Neural Network
      mask Display: e = 0.06;c1 = [120 150 230]/255;c2 = ([120 150 230]+0)/383;c3 = ([120 150 230]+128)/383;patch([0 1 1 0],[0 0 1 1],c1);patch([0 1 1 1-e 1-e 0+e],[0 0 1 1-e 0+e 0+e],c2);patch([0 0 1 1-e 0+e 0+e],[0 1 1 1-e 1-e 0+e],c3);plot([0 1 1 0 0],[0 0 1 1 0]);fprintf('NNET');port_label('input',1,' Input');port_label('output',1,'Output ');
  Hue_adjusted : Display
  K : Display
  Mux : Mux
  R : Display
  RGB to HSV : MATLAB Function  TreatAsAtomicUnit=on
  Sat Neural Network : Subsystem
      mask help: Feed-Forward Neural Network
      mask Display: e = 0.06;c1 = [120 150 230]/255;c2 = ([120 150 230]+0)/383;c3 = ([120 150 230]+128)/383;patch([0 1 1 0],[0 0 1 1],c1);patch([0 1 1 1-e 1-e 0+e],[0 0 1 1-e 0+e 0+e],c2);patch([0 0 1 1-e 0+e 0+e],[0 1 1 1-e 1-e 0+e],c3);plot([0 1 1 0 0],[0 0 1 1 0]);fprintf('NNET');port_label('input',1,' Input');port_label('output',1,'Output ');
  Saturation_adjusted : Display
  hue_post_processor : MATLAB Function  TreatAsAtomicUnit=on
  sat_post_processor : MATLAB Function  TreatAsAtomicUnit=on
  sat_post_processor1 : MATLAB Function  TreatAsAtomicUnit=on
  Hue : Outport
  Sat : Outport  Port=2
  wires:
  red/1 -> R/1, RGB to HSV/1("R ")  "red"
  green/1 -> G/1, RGB to HSV/2("G ")  "green"
  blue/1 -> B/1, RGB to HSV/3("B ")  "blue"
  greyscale/1 -> K/1, RGB to HSV/4("K ")
  RGB to HSV/4(K) -> Mux/4
  RGB to HSV/3(B) -> Mux/3
  RGB to HSV/2(G) -> Mux/2
  RGB to HSV/1(R) -> Mux/1
  hue_post_processor/1(hue) -> Hue_adjusted/1, Hue/1
  sat_post_processor/1(sat) -> Sat/1, Saturation_adjusted/1
  Hue Neural Network/1(Output) -> Demux/1
  Demux/1 -> hue_post_processor/1(hue_nn_sin)
  Demux/2 -> hue_post_processor/2(hue_nn_cos)
  sat_post_processor1/1(data) -> Hue Neural Network/1(Input), Sat Neural Network/1(Input)
  Mux/1 -> sat_post_processor1/1(data_raw)
  Sat Neural Network/1(Output) -> sat_post_processor/1(sat_nn_output)

== system chris_4R_all_primitives/RGB to HSV to vel - all robots4 ==
  greyscale : Inport
  red : Inport  Port=2
  green : Inport  Port=3
  blue : Inport  Port=4
  B : Display
  Demux : Demux  Outputs=2
  G : Display
  Hue Neural Network : Subsystem
      mask help: Feed-Forward Neural Network
      mask Display: e = 0.06;c1 = [120 150 230]/255;c2 = ([120 150 230]+0)/383;c3 = ([120 150 230]+128)/383;patch([0 1 1 0],[0 0 1 1],c1);patch([0 1 1 1-e 1-e 0+e],[0 0 1 1-e 0+e 0+e],c2);patch([0 0 1 1-e 0+e 0+e],[0 1 1 1-e 1-e 0+e],c3);plot([0 1 1 0 0],[0 0 1 1 0]);fprintf('NNET');port_label('input',1,' Input');port_label('output',1,'Output ');
  Hue_adjusted : Display
  K : Display
  Mux : Mux
  R : Display
  RGB to HSV : MATLAB Function  TreatAsAtomicUnit=on
  Sat Neural Network : Subsystem
      mask help: Feed-Forward Neural Network
      mask Display: e = 0.06;c1 = [120 150 230]/255;c2 = ([120 150 230]+0)/383;c3 = ([120 150 230]+128)/383;patch([0 1 1 0],[0 0 1 1],c1);patch([0 1 1 1-e 1-e 0+e],[0 0 1 1-e 0+e 0+e],c2);patch([0 0 1 1-e 0+e 0+e],[0 1 1 1-e 1-e 0+e],c3);plot([0 1 1 0 0],[0 0 1 1 0]);fprintf('NNET');port_label('input',1,' Input');port_label('output',1,'Output ');
  Saturation_adjusted : Display
  hue_post_processor : MATLAB Function  TreatAsAtomicUnit=on
  sat_post_processor : MATLAB Function  TreatAsAtomicUnit=on
  sat_post_processor1 : MATLAB Function  TreatAsAtomicUnit=on
  Hue : Outport
  Sat : Outport  Port=2
  wires:
  red/1 -> R/1, RGB to HSV/1("R ")  "red"
  green/1 -> G/1, RGB to HSV/2("G ")  "green"
  blue/1 -> B/1, RGB to HSV/3("B ")  "blue"
  greyscale/1 -> K/1, RGB to HSV/4("K ")
  RGB to HSV/4(K) -> Mux/4
  RGB to HSV/3(B) -> Mux/3
  RGB to HSV/2(G) -> Mux/2
  RGB to HSV/1(R) -> Mux/1
  hue_post_processor/1(hue) -> Hue_adjusted/1, Hue/1
  sat_post_processor/1(sat) -> Sat/1, Saturation_adjusted/1
  Hue Neural Network/1(Output) -> Demux/1
  Demux/1 -> hue_post_processor/1(hue_nn_sin)
  Demux/2 -> hue_post_processor/2(hue_nn_cos)
  sat_post_processor1/1(data) -> Hue Neural Network/1(Input), Sat Neural Network/1(Input)
  Mux/1 -> sat_post_processor1/1(data_raw)
  Sat Neural Network/1(Output) -> sat_post_processor/1(sat_nn_output)

== system chris_4R_all_primitives/Robot_signal_processing_1 ==
  Optitrack_in : Inport
  velocity_in : Inport  Port=2
  Demux4 : Demux  Outputs=3
  Global to Body Velocities : Product  Multiplication=Matrix(*)
  Global to Body Rotation Matrix : MATLAB Function  TreatAsAtomicUnit=on
  Math Function : Math  Operator=transpose  SignedPower=on
  Mux : Mux  Inputs=3
  Signal_Reshape : Reshape  OutputDimensions=6
  Signal_Select : Selector  InputPortWidth=6  IndexOptions=Index vector (dialog)  Indices=[1 2 6]  OutputSizes=1
  To Workspace : ToWorkspace  VariableName=robot1_pose  SampleTime=-1
  Processed_Signal : Outport
  XZTH_Mux : Outport  Port=2
  wires:
  Demux4/3 -> Mux/3, Global to Body Rotation Matrix/1(u)  "theta"
  Global to Body Velocities/1 -> Processed_Signal/1
  Signal_Reshape/1 -> Signal_Select/1
  velocity_in/1 -> Global to Body Velocities/2
  Optitrack_in/1 -> Signal_Reshape/1
  Global to Body Rotation Matrix/1(y) -> Math Function/1
  Math Function/1 -> Global to Body Velocities/1
  Signal_Select/1 -> To Workspace/1, Demux4/1
  Mux/1 -> XZTH_Mux/1
  Demux4/2 -> Mux/2  "Z"
  Demux4/1 -> Mux/1  "X"

== system chris_4R_all_primitives/Robot_signal_processing_2 ==
  Optitrack_in : Inport
  velocity_in : Inport  Port=2
  Demux4 : Demux  Outputs=3
  Global to Body Velocities : Product  Multiplication=Matrix(*)
  Global to Body Rotation Matrix : MATLAB Function  TreatAsAtomicUnit=on
  Math Function : Math  Operator=transpose  SignedPower=on
  Mux : Mux  Inputs=3
  Signal_Reshape : Reshape  OutputDimensions=6
  Signal_Select : Selector  InputPortWidth=6  IndexOptions=Index vector (dialog)  Indices=[1 2 6]  OutputSizes=1
  To Workspace : ToWorkspace  VariableName=robot2_pose  SampleTime=-1
  Processed_Signal : Outport
  XZTH_Mux : Outport  Port=2
  wires:
  Demux4/1 -> Mux/1  "X"
  Demux4/3 -> Mux/3, Global to Body Rotation Matrix/1(u)  "theta"
  Demux4/2 -> Mux/2  "Z"
  Global to Body Velocities/1 -> Processed_Signal/1
  Signal_Reshape/1 -> Signal_Select/1
  velocity_in/1 -> Global to Body Velocities/2
  Optitrack_in/1 -> Signal_Reshape/1
  Global to Body Rotation Matrix/1(y) -> Math Function/1
  Signal_Select/1 -> To Workspace/1, Demux4/1
  Math Function/1 -> Global to Body Velocities/1
  Mux/1 -> XZTH_Mux/1

== system chris_4R_all_primitives/Robot_signal_processing_3 ==
  Optitrack_in : Inport
  velocity_in : Inport  Port=2
  Demux4 : Demux  Outputs=3
  Global to Body Velocities : Product  Multiplication=Matrix(*)
  Global to Body Rotation Matrix : MATLAB Function  TreatAsAtomicUnit=on
  Math Function : Math  Operator=transpose  SignedPower=on
  Mux : Mux  Inputs=3
  Signal_Reshape : Reshape  OutputDimensions=6
  Signal_Select : Selector  InputPortWidth=6  IndexOptions=Index vector (dialog)  Indices=[1 2 6]  OutputSizes=1
  To Workspace : ToWorkspace  VariableName=robot3_pose  SampleTime=-1
  Processed_Signal : Outport
  XZTH_Mux : Outport  Port=2
  wires:
  Demux4/1 -> Mux/1  "X"
  Demux4/3 -> Mux/3, Global to Body Rotation Matrix/1(u)  "theta"
  Demux4/2 -> Mux/2  "Z"
  Global to Body Velocities/1 -> Processed_Signal/1
  Signal_Reshape/1 -> Signal_Select/1
  velocity_in/1 -> Global to Body Velocities/2
  Optitrack_in/1 -> Signal_Reshape/1
  Global to Body Rotation Matrix/1(y) -> Math Function/1
  Signal_Select/1 -> Demux4/1
  Math Function/1 -> Global to Body Velocities/1
  Mux/1 -> To Workspace/1, XZTH_Mux/1

== system chris_4R_all_primitives/Robot_signal_processing_4 ==
  Optitrack_in : Inport
  velocity_in : Inport  Port=2
  Demux4 : Demux  Outputs=3
  Global to Body Velocities : Product  Multiplication=Matrix(*)
  Global to Body Rotation Matrix : MATLAB Function  TreatAsAtomicUnit=on
  Math Function : Math  Operator=transpose  SignedPower=on
  Mux : Mux  Inputs=3
  Signal_Reshape : Reshape  OutputDimensions=6
  Signal_Select : Selector  InputPortWidth=6  IndexOptions=Index vector (dialog)  Indices=[1 2 6]  OutputSizes=1
  To Workspace : ToWorkspace  VariableName=robot4_pose  SampleTime=-1
  Processed_Signal : Outport
  XZTH_Mux : Outport  Port=2
  wires:
  Demux4/1 -> Mux/1  "X"
  Demux4/3 -> Mux/3, Global to Body Rotation Matrix/1(u)  "theta"
  Demux4/2 -> Mux/2  "Z"
  Global to Body Velocities/1 -> Processed_Signal/1
  Signal_Reshape/1 -> Signal_Select/1
  velocity_in/1 -> Global to Body Velocities/2
  Optitrack_in/1 -> Signal_Reshape/1
  Global to Body Rotation Matrix/1(y) -> Math Function/1
  Signal_Select/1 -> Demux4/1
  Math Function/1 -> Global to Body Velocities/1
  Mux/1 -> To Workspace/1, XZTH_Mux/1

== system chris_4R_all_primitives/celeste ==
  In1 : Inport
  In2 : Inport  Port=2
  In3 : Inport  Port=3
  Signal Specification : SignalSpecification  OutDataTypeStr=double  Dimensions=1
  Signal Specification1 : SignalSpecification  OutDataTypeStr=double  Dimensions=1
  Signal Specification2 : SignalSpecification  OutDataTypeStr=double  Dimensions=1
  decabot : MATLABSystem  System=Decabot  robotName=celeste  decabotHelper=localhost  useDataTurbine=off  useDirectSocket=on  debug=off
      mask Type: Decabot
      mask Display:
      | disp('celeste\n\nDH: localhost');
      | port_label('input',1,'x_vel');
      | port_label('input',2,'y_vel');
      | port_label('input',3,'t_vel');
      | port_label('output',1,'clear');
      | port_label('output',2,'red');
      | port_label('output',3,'green');
      | port_label('output',4,'blue');
  Out1 : Outport
  Out2 : Outport  Port=2
  Out3 : Outport  Port=3
  Out4 : Outport  Port=4
  wires:
  Signal Specification2/1 -> decabot/3
  Signal Specification1/1 -> decabot/2
  Signal Specification/1 -> decabot/1
  In2/1 -> Signal Specification1/1
  decabot/4 -> Out4/1
  decabot/1 -> Out1/1
  decabot/3 -> Out3/1
  decabot/2 -> Out2/1
  In1/1 -> Signal Specification/1
  In3/1 -> Signal Specification2/1

== system chris_4R_all_primitives/pacific-blue ==
  In1 : Inport
  In2 : Inport  Port=2
  In3 : Inport  Port=3
  Signal Specification : SignalSpecification  OutDataTypeStr=double  Dimensions=1
  Signal Specification1 : SignalSpecification  OutDataTypeStr=double  Dimensions=1
  Signal Specification2 : SignalSpecification  OutDataTypeStr=double  Dimensions=1
  decabot : MATLABSystem  System=Decabot  robotName=pacific-blue  decabotHelper=localhost  useDataTurbine=off  useDirectSocket=on  debug=off
      mask Type: Decabot
      mask Display:
      | disp('pacific-blue\n\nDH: localhost');
      | port_label('input',1,'x_vel');
      | port_label('input',2,'y_vel');
      | port_label('input',3,'t_vel');
      | port_label('output',1,'clear');
      | port_label('output',2,'red');
      | port_label('output',3,'green');
      | port_label('output',4,'blue');
  Out1 : Outport
  Out2 : Outport  Port=2
  Out3 : Outport  Port=3
  Out4 : Outport  Port=4
  wires:
  Signal Specification2/1 -> decabot/3
  Signal Specification1/1 -> decabot/2
  Signal Specification/1 -> decabot/1
  In2/1 -> Signal Specification1/1
  decabot/4 -> Out4/1
  decabot/1 -> Out1/1
  decabot/3 -> Out3/1
  decabot/2 -> Out2/1
  In1/1 -> Signal Specification/1
  In3/1 -> Signal Specification2/1

== system chris_4R_all_primitives/redwood ==
  In1 : Inport
  In2 : Inport  Port=2
  In3 : Inport  Port=3
  Signal Specification : SignalSpecification  OutDataTypeStr=double  Dimensions=1
  Signal Specification1 : SignalSpecification  OutDataTypeStr=double  Dimensions=1
  Signal Specification2 : SignalSpecification  OutDataTypeStr=double  Dimensions=1
  decabot : MATLABSystem  System=Decabot  robotName=redwood  decabotHelper=localhost  useDataTurbine=off  useDirectSocket=on  debug=off
      mask Type: Decabot
      mask Display:
      | disp('redwood\n\nDH: localhost');
      | port_label('input',1,'x_vel');
      | port_label('input',2,'y_vel');
      | port_label('input',3,'t_vel');
      | port_label('output',1,'clear');
      | port_label('output',2,'red');
      | port_label('output',3,'green');
      | port_label('output',4,'blue');
  Out1 : Outport
  Out2 : Outport  Port=2
  Out3 : Outport  Port=3
  Out4 : Outport  Port=4
  wires:
  Signal Specification2/1 -> decabot/3
  Signal Specification1/1 -> decabot/2
  Signal Specification/1 -> decabot/1
  In2/1 -> Signal Specification1/1
  decabot/4 -> Out4/1
  decabot/1 -> Out1/1
  decabot/3 -> Out3/1
  decabot/2 -> Out2/1
  In1/1 -> Signal Specification/1
  In3/1 -> Signal Specification2/1
